simulink model "Plant"  (R2023a)
settings: Solver=VariableStepAuto  StartTime=0.0  StopTime=10.0  RelTol=1e-3
undefined symbols (not defined in the file): c, C, C1, C2, C_alpha_f, C_r, E, e_p0, F_zf, Iz, J1, J2, K, l_f, l_r, m, n_st, T_f
settings Model: Creator=Tan_Tram  LastModifiedBy=Tan_Tram

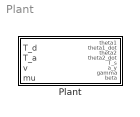
== system Plant ==
  Plant : Subsystem

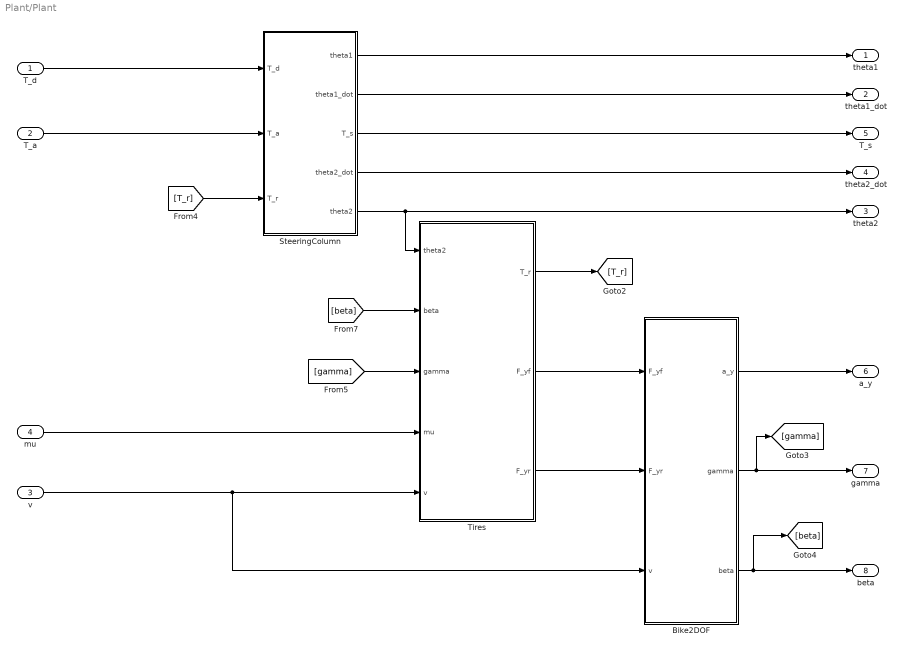
== system Plant/Plant ==
  T_d : Inport
  T_a : Inport  Port=2
  v : Inport  Port=3
  mu : Inport  Port=4
  Bike2DOF : Subsystem
  SteeringColumn : Subsystem
  Tires : Subsystem
  theta1 : Outport
  theta1_dot : Outport  Port=2
  theta2 : Outport  Port=3
  theta2_dot : Outport  Port=4
  T_s : Outport  Port=5
  a_y : Outport  Port=6
  gamma : Outport  Port=7
  beta : Outport  Port=8
  wires:
  [beta] -> Tires/2(beta)
  T_d/1 -> SteeringColumn/1(T_d)
  [T_r] -> SteeringColumn/3(T_r)
  Bike2DOF/3(beta) -> beta/1, [beta]
  T_a/1 -> SteeringColumn/2(T_a)
  Tires/1(T_r) -> [T_r]
  SteeringColumn/5(theta2) -> theta2/1, Tires/1(theta2)
  [gamma] -> Tires/3(gamma)
  Tires/3(F_yr) -> Bike2DOF/2(F_yr)
  mu/1 -> Tires/4(mu)
  SteeringColumn/1(theta1) -> theta1/1
  Bike2DOF/2(gamma) -> [gamma], gamma/1
  SteeringColumn/2(theta1_dot) -> theta1_dot/1
  SteeringColumn/3(T_s) -> T_s/1
  SteeringColumn/4(theta2_dot) -> theta2_dot/1
  Tires/2(F_yf) -> Bike2DOF/1(F_yf)
  v/1 -> Bike2DOF/3(v), Tires/5(v)
  Bike2DOF/1(a_y) -> a_y/1

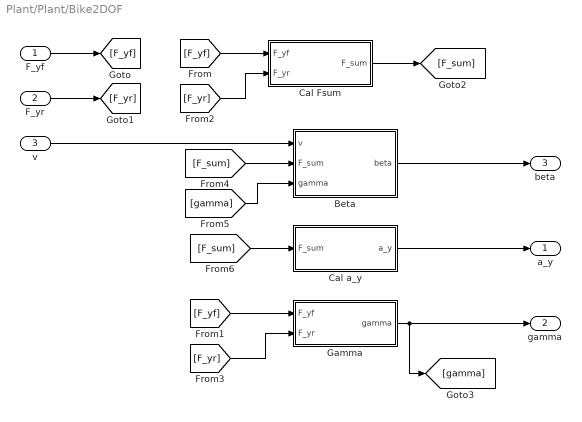
== system Plant/Plant/Bike2DOF ==
  F_yf : Inport
  F_yr : Inport  Port=2
  v : Inport  Port=3
  Beta : Subsystem
  Cal Fsum : Subsystem
  Cal a_y : Subsystem
  Gamma : Subsystem
  a_y : Outport
  gamma : Outport  Port=2
  beta : Outport  Port=3
  wires:
  [F_sum] -> Cal a_y/1(F_sum)
  Cal a_y/1(a_y) -> a_y/1
  Cal Fsum/1(F_sum) -> [F_sum]
  Beta/1(beta) -> beta/1
  [F_yr] -> Gamma/2(F_yr)
  [F_yf] -> Gamma/1(F_yf)
  [gamma] -> Beta/3(gamma)
  [F_yr] -> Cal Fsum/2(F_yr)
  v/1 -> Beta/1(v)
  F_yf/1 -> [F_yf]
  Gamma/1(gamma) -> [gamma], gamma/1
  [F_sum] -> Beta/2(F_sum)
  [F_yf] -> Cal Fsum/1(F_yf)
  F_yr/1 -> [F_yr]

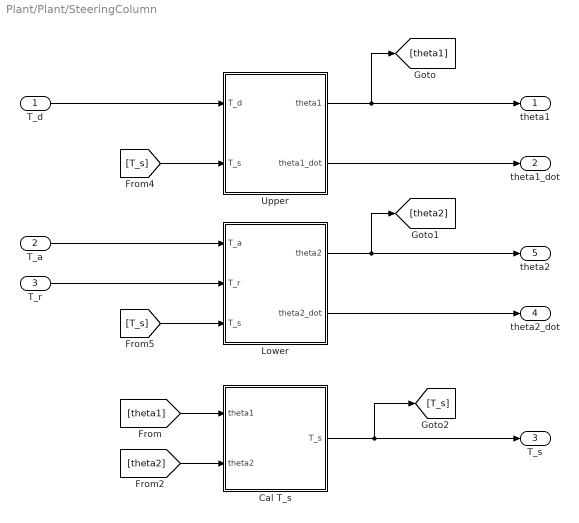
== system Plant/Plant/SteeringColumn ==
  T_d : Inport
  T_a : Inport  Port=2
  T_r : Inport  Port=3
  Cal T_s : Subsystem
  Lower : Subsystem
  Upper : Subsystem
  theta1 : Outport
  theta1_dot : Outport  Port=2
  T_s : Outport  Port=3
  theta2_dot : Outport  Port=4
  theta2 : Outport  Port=5
  wires:
  Lower/2(theta2_dot) -> theta2_dot/1
  Upper/2(theta1_dot) -> theta1_dot/1
  Cal T_s/1(T_s) -> [T_s], T_s/1
  [T_s] -> Lower/3(T_s)
  [T_s] -> Upper/2(T_s)
  Lower/1(theta2) -> [theta2], theta2/1
  [theta2] -> Cal T_s/2(theta2)
  Upper/1(theta1) -> [theta1], theta1/1
  [theta1] -> Cal T_s/1(theta1)
  T_r/1 -> Lower/2(T_r)
  T_a/1 -> Lower/1(T_a)
  T_d/1 -> Upper/1(T_d)

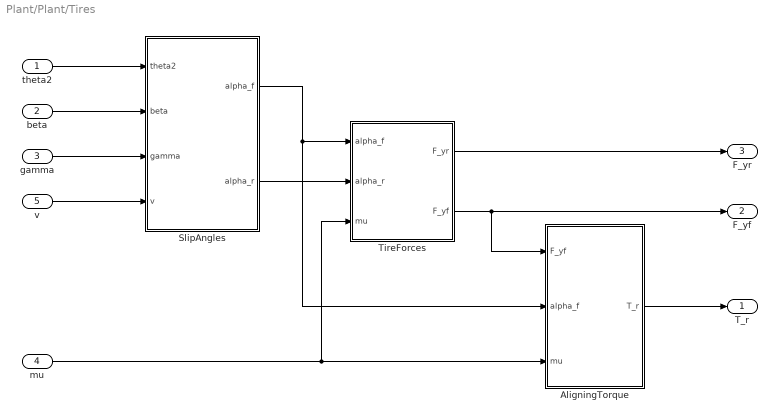
== system Plant/Plant/Tires ==
  theta2 : Inport
  beta : Inport  Port=2
  gamma : Inport  Port=3
  mu : Inport  Port=4
  v : Inport  Port=5
  AligningTorque : Subsystem
  SlipAngles : Subsystem
  TireForces : Subsystem
  T_r : Outport
  F_yf : Outport  Port=2
  F_yr : Outport  Port=3
  wires:
  AligningTorque/1(T_r) -> T_r/1
  TireForces/1(F_yr) -> F_yr/1
  mu/1 -> TireForces/3(mu), AligningTorque/3(mu)
  SlipAngles/1(alpha_f) -> AligningTorque/2(alpha_f), TireForces/1(alpha_f)
  SlipAngles/2(alpha_r) -> TireForces/2(alpha_r)
  theta2/1 -> SlipAngles/1(theta2)
  beta/1 -> SlipAngles/2(beta)
  TireForces/2(F_yf) -> AligningTorque/1(F_yf), F_yf/1
  gamma/1 -> SlipAngles/3(gamma)
  v/1 -> SlipAngles/4(v)

== system Plant/Plant/Bike2DOF/Beta ==
  v : Inport
  F_sum : Inport  Port=2
  gamma : Inport  Port=3
  Constant : Constant  Value=m
  Div_Fsum_mv : Product  Inputs=*/
  Int_beta : Integrator
  Prod_mv : Product  Inputs=**
  Sum_betadot : Sum  Inputs=+-
  beta : Outport
  wires:
  gamma/1 -> Sum_betadot/2
  Prod_mv/1 -> Div_Fsum_mv/2
  F_sum/1 -> Div_Fsum_mv/1
  Div_Fsum_mv/1 -> Sum_betadot/1
  v/1 -> Prod_mv/2
  Int_beta/1 -> beta/1
  Constant/1 -> Prod_mv/1
  Sum_betadot/1 -> Int_beta/1

== system Plant/Plant/Bike2DOF/Cal Fsum ==
  F_yf : Inport
  F_yr : Inport  Port=2
  Sum_Fsum : Sum
  F_sum : Outport
  wires:
  Sum_Fsum/1 -> F_sum/1
  F_yf/1 -> Sum_Fsum/1
  F_yr/1 -> Sum_Fsum/2

== system Plant/Plant/Bike2DOF/Cal a_y ==
  F_sum : Inport
  Constant : Constant  Value=m
  Div_ay : Product  Inputs=*/
  a_y : Outport
  wires:
  F_sum/1 -> Div_ay/1
  Constant/1 -> Div_ay/2
  Div_ay/1 -> a_y/1

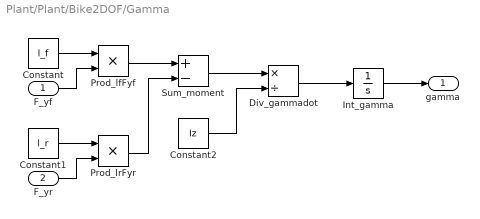
== system Plant/Plant/Bike2DOF/Gamma ==
  F_yf : Inport
  F_yr : Inport  Port=2
  Constant : Constant  Value=l_f
  Constant1 : Constant  Value=l_r
  Constant2 : Constant  Value=Iz
  Div_gammadot : Product  Inputs=*/
  Int_gamma : Integrator
  Prod_lfFyf : Product  Inputs=**
  Prod_lrFyr : Product  Inputs=**
  Sum_moment : Sum  Inputs=+-
  gamma : Outport
  wires:
  Div_gammadot/1 -> Int_gamma/1
  Sum_moment/1 -> Div_gammadot/1
  Prod_lrFyr/1 -> Sum_moment/2
  Constant2/1 -> Div_gammadot/2
  F_yr/1 -> Prod_lrFyr/2
  Constant1/1 -> Prod_lrFyr/1
  Int_gamma/1 -> gamma/1
  Constant/1 -> Prod_lfFyf/1
  F_yf/1 -> Prod_lfFyf/2
  Prod_lfFyf/1 -> Sum_moment/1

== system Plant/Plant/SteeringColumn/Cal T_s ==
  theta1 : Inport
  theta2 : Inport  Port=2
  Constant : Constant  Value=K
  Prod_Ts : Product  Inputs=**
  Sum_dTheta : Sum  Inputs=+-
  T_s : Outport
  wires:
  theta2/1 -> Sum_dTheta/2
  Prod_Ts/1 -> T_s/1
  theta1/1 -> Sum_dTheta/1
  Sum_dTheta/1 -> Prod_Ts/1
  Constant/1 -> Prod_Ts/2

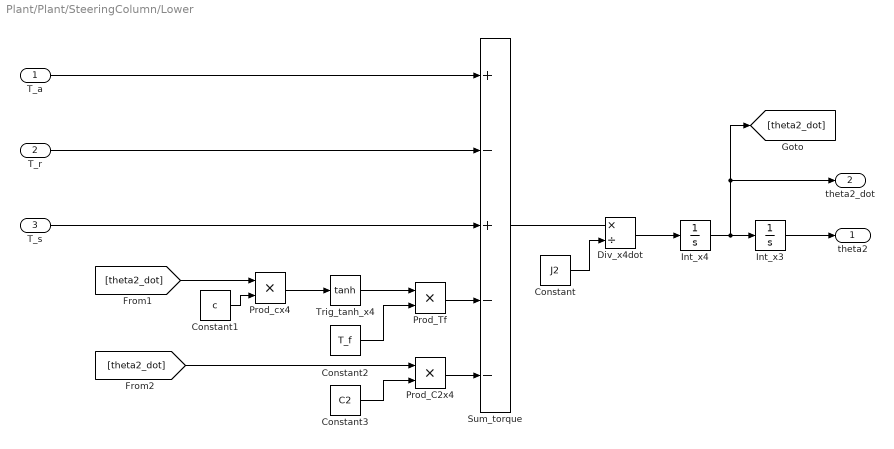
== system Plant/Plant/SteeringColumn/Lower ==
  T_a : Inport
  T_r : Inport  Port=2
  T_s : Inport  Port=3
  Constant : Constant  Value=J2
  Constant1 : Constant  Value=c
  Constant2 : Constant  Value=T_f
  Constant3 : Constant  Value=C2
  Div_x4dot : Product  Inputs=*/
  Int_x3 : Integrator
  Int_x4 : Integrator
  Prod_C2x4 : Product  Inputs=**
  Prod_Tf : Product  Inputs=**
  Prod_cx4 : Product  Inputs=**
  Sum_torque : Sum  Inputs=+-+--
  Trig_tanh_x4 : Trigonometry  Operator=tanh
  theta2 : Outport
  theta2_dot : Outport  Port=2
  wires:
  Div_x4dot/1 -> Int_x4/1
  Constant/1 -> Div_x4dot/2
  Sum_torque/1 -> Div_x4dot/1
  Prod_Tf/1 -> Sum_torque/4
  T_s/1 -> Sum_torque/3
  T_a/1 -> Sum_torque/1
  Constant3/1 -> Prod_C2x4/2
  Prod_C2x4/1 -> Sum_torque/5
  [theta2_dot] -> Prod_C2x4/1
  Trig_tanh_x4/1 -> Prod_Tf/1
  Prod_cx4/1 -> Trig_tanh_x4/1
  Constant1/1 -> Prod_cx4/2
  Int_x4/1 -> Int_x3/1, theta2_dot/1, [theta2_dot]
  [theta2_dot] -> Prod_cx4/1
  Int_x3/1 -> theta2/1
  T_r/1 -> Sum_torque/2
  Constant2/1 -> Prod_Tf/2

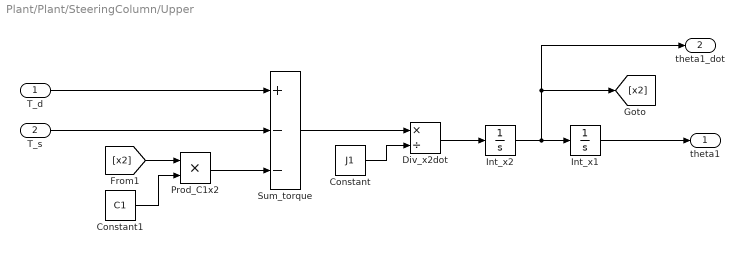
== system Plant/Plant/SteeringColumn/Upper ==
  T_d : Inport
  T_s : Inport  Port=2
  Constant : Constant  Value=J1
  Constant1 : Constant  Value=C1
  Div_x2dot : Product  Inputs=*/
  Int_x1 : Integrator
  Int_x2 : Integrator
  Prod_C1x2 : Product  Inputs=**
  Sum_torque : Sum  Inputs=+--
  theta1 : Outport
  theta1_dot : Outport  Port=2
  wires:
  Div_x2dot/1 -> Int_x2/1
  Constant/1 -> Div_x2dot/2
  T_s/1 -> Sum_torque/2
  [x2] -> Prod_C1x2/1
  Int_x1/1 -> theta1/1
  Prod_C1x2/1 -> Sum_torque/3
  Int_x2/1 -> [x2], theta1_dot/1, Int_x1/1
  Constant1/1 -> Prod_C1x2/2
  Sum_torque/1 -> Div_x2dot/1
  T_d/1 -> Sum_torque/1

== system Plant/Plant/Tires/AligningTorque ==
  F_yf : Inport
  alpha_f : Inport  Port=2
  mu : Inport  Port=3
  K_tr : Subsystem
  Prod_Tr : Product  Inputs=**
  e_p : Subsystem
  T_r : Outport
  wires:
  K_tr/1(K_tr) -> Prod_Tr/1
  e_p/1(e_p) -> K_tr/1(e_p)
  mu/1 -> e_p/2(mu)
  alpha_f/1 -> e_p/1(alpha_f)
  Prod_Tr/1 -> T_r/1
  F_yf/1 -> Prod_Tr/2

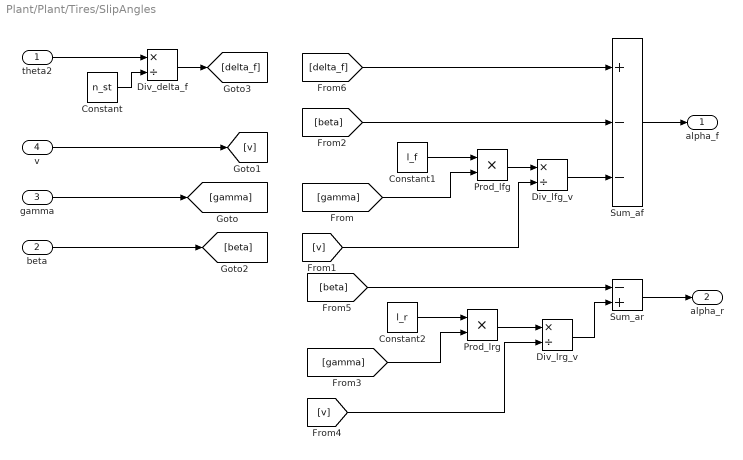
== system Plant/Plant/Tires/SlipAngles ==
  theta2 : Inport
  beta : Inport  Port=2
  gamma : Inport  Port=3
  v : Inport  Port=4
  Constant : Constant  Value=n_st
  Constant1 : Constant  Value=l_f
  Constant2 : Constant  Value=l_r
  Div_delta_f : Product  Inputs=*/
  Div_lfg_v : Product  Inputs=*/
  Div_lrg_v : Product  Inputs=*/
  Prod_lfg : Product  Inputs=**
  Prod_lrg : Product  Inputs=**
  Sum_af : Sum  Inputs=+--
  Sum_ar : Sum  Inputs=-+
  alpha_f : Outport
  alpha_r : Outport  Port=2
  wires:
  theta2/1 -> Div_delta_f/1
  Constant/1 -> Div_delta_f/2
  Div_delta_f/1 -> [delta_f]
  [delta_f] -> Sum_af/1
  [beta] -> Sum_ar/1
  [beta] -> Sum_af/2
  Sum_af/1 -> alpha_f/1
  Prod_lrg/1 -> Div_lrg_v/1
  [v] -> Div_lfg_v/2
  Prod_lfg/1 -> Div_lfg_v/1
  [v] -> Div_lrg_v/2
  Sum_ar/1 -> alpha_r/1
  [gamma] -> Prod_lrg/2
  v/1 -> [v]
  [gamma] -> Prod_lfg/2
  gamma/1 -> [gamma]
  Constant1/1 -> Prod_lfg/1
  Div_lfg_v/1 -> Sum_af/3
  Constant2/1 -> Prod_lrg/1
  Div_lrg_v/1 -> Sum_ar/2
  beta/1 -> [beta]

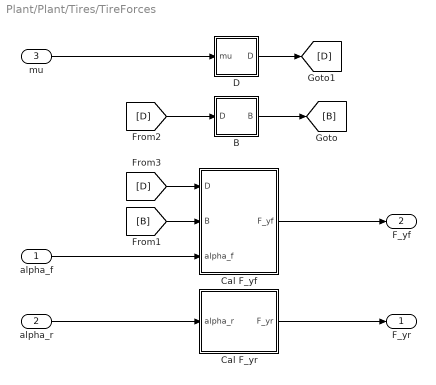
== system Plant/Plant/Tires/TireForces ==
  alpha_f : Inport
  alpha_r : Inport  Port=2
  mu : Inport  Port=3
  B : Subsystem
  Cal F_yf : Subsystem
  Cal F_yr : Subsystem
  D : Subsystem
  F_yr : Outport
  F_yf : Outport  Port=2
  wires:
  [D] -> Cal F_yf/1(D)
  [B] -> Cal F_yf/2(B)
  Cal F_yf/1(F_yf) -> F_yf/1
  alpha_f/1 -> Cal F_yf/3(alpha_f)
  B/1(B) -> [B]
  Cal F_yr/1(F_yr) -> F_yr/1
  alpha_r/1 -> Cal F_yr/1(alpha_r)
  [D] -> B/1(D)
  D/1(D) -> [D]
  mu/1 -> D/1(mu)

== system Plant/Plant/Tires/AligningTorque/K_tr ==
  e_p : Inport
  Constant4 : Constant  Value=n_st
  Div_Ktr : Product  Inputs=*/
  K_tr : Outport
  wires:
  Constant4/1 -> Div_Ktr/2
  e_p/1 -> Div_Ktr/1
  Div_Ktr/1 -> K_tr/1

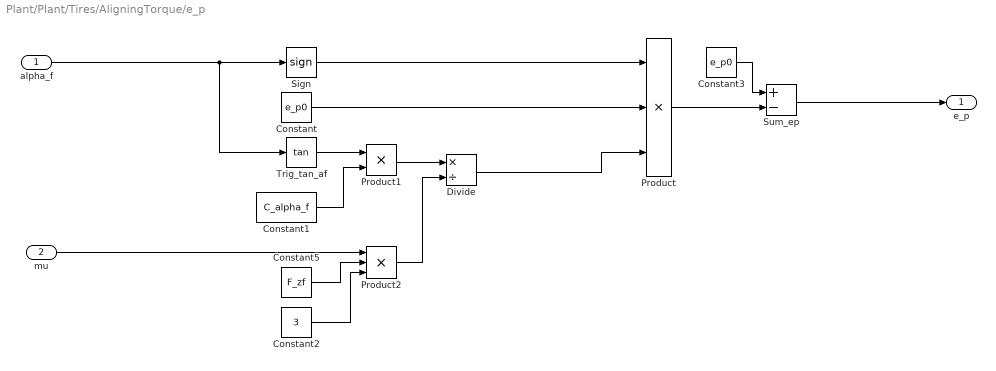
== system Plant/Plant/Tires/AligningTorque/e_p ==
  alpha_f : Inport
  mu : Inport  Port=2
  Constant : Constant  Value=e_p0
  Constant1 : Constant  Value=C_alpha_f
  Constant2 : Constant  Value=3
  Constant3 : Constant  Value=e_p0
  Constant5 : Constant  Value=F_zf
  Divide : Product  Inputs=*/
  Product : Product  Inputs=3
  Product1 : Product
  Product2 : Product  Inputs=***
  Sign : Signum
  Sum_ep : Sum  Inputs=+-
  Trig_tan_af : Trigonometry  Operator=tan
  e_p : Outport
  wires:
  Sum_ep/1 -> e_p/1
  Sign/1 -> Product/1
  Product2/1 -> Divide/2
  Divide/1 -> Product/3
  Constant2/1 -> Product2/3
  Product/1 -> Sum_ep/2
  Constant3/1 -> Sum_ep/1
  Constant5/1 -> Product2/2
  Trig_tan_af/1 -> Product1/1
  mu/1 -> Product2/1
  Constant1/1 -> Product1/2
  alpha_f/1 -> Trig_tan_af/1, Sign/1
  Product1/1 -> Divide/1
  Constant/1 -> Product/2

== system Plant/Plant/Tires/TireForces/B ==
  D : Inport
  Constant : Constant  Value=C
  Constant1 : Constant  Value=C_alpha_f
  Div_B : Product  Inputs=*/
  Prod_CD : Product  Inputs=**
  B : Outport
  wires:
  D/1 -> Prod_CD/2
  Constant/1 -> Prod_CD/1
  Constant1/1 -> Div_B/1
  Prod_CD/1 -> Div_B/2
  Div_B/1 -> B/1

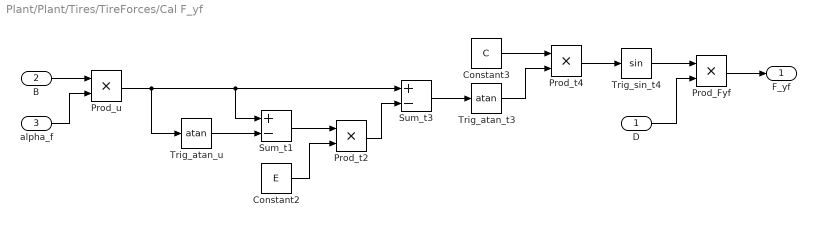
== system Plant/Plant/Tires/TireForces/Cal F_yf ==
  D : Inport
  B : Inport  Port=2
  alpha_f : Inport  Port=3
  Constant2 : Constant  Value=E
  Constant3 : Constant  Value=C
  Prod_Fyf : Product  Inputs=**
  Prod_t2 : Product  Inputs=**
  Prod_t4 : Product  Inputs=**
  Prod_u : Product  Inputs=**
  Sum_t1 : Sum  Inputs=+-
  Sum_t3 : Sum  Inputs=+-
  Trig_atan_t3 : Trigonometry  Operator=atan
  Trig_atan_u : Trigonometry  Operator=atan
  Trig_sin_t4 : Trigonometry
  F_yf : Outport
  wires:
  D/1 -> Prod_Fyf/2
  Prod_t4/1 -> Trig_sin_t4/1
  Constant3/1 -> Prod_t4/1
  Trig_atan_u/1 -> Sum_t1/2
  Constant2/1 -> Prod_t2/2
  Prod_Fyf/1 -> F_yf/1
  Prod_u/1 -> Trig_atan_u/1, Sum_t3/1, Sum_t1/1
  Trig_atan_t3/1 -> Prod_t4/2
  Prod_t2/1 -> Sum_t3/2
  Sum_t1/1 -> Prod_t2/1
  Trig_sin_t4/1 -> Prod_Fyf/1
  Sum_t3/1 -> Trig_atan_t3/1
  B/1 -> Prod_u/1
  alpha_f/1 -> Prod_u/2

== system Plant/Plant/Tires/TireForces/Cal F_yr ==
  alpha_r : Inport
  Constant4 : Constant  Value=C_r
  Prod_Fyr : Product  Inputs=**
  F_yr : Outport
  wires:
  alpha_r/1 -> Prod_Fyr/2
  Prod_Fyr/1 -> F_yr/1
  Constant4/1 -> Prod_Fyr/1

== system Plant/Plant/Tires/TireForces/D ==
  mu : Inport
  Constant7 : Constant  Value=F_zf
  Prod_D : Product  Inputs=**
  D : Outport
  wires:
  Constant7/1 -> Prod_D/2
  Prod_D/1 -> D/1
  mu/1 -> Prod_D/1
